simulink model "architecture"  (R2019a)
settings: Solver=VariableStepAuto  StartTime=0.0  StopTime=10.0  RelTol=1e-3
settings Model: Creator=gustavo.nunes  LastModifiedBy=gustavo.nunes

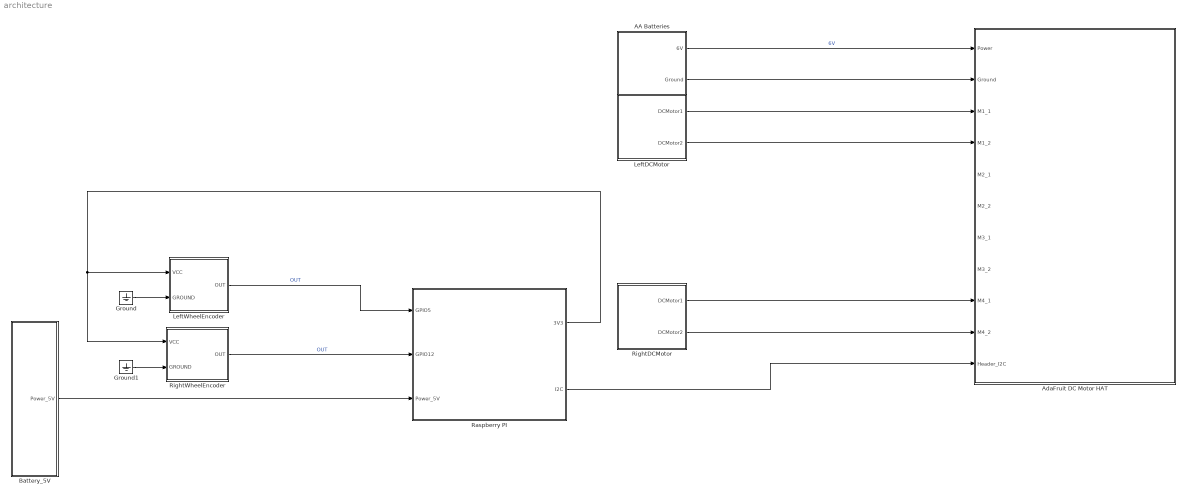
== system architecture ==
  AA Batteries : Subsystem
      mask Display: image('aa_battery.png');
  AdaFruit DC Motor HAT : Subsystem
  Battery_5V : Subsystem
      mask Display: image('battery.png');
  Ground : Ground
  Ground1 : Ground
  LeftDCMotor : Subsystem
      mask Display: image('tt_dc_motor.png');
  LeftWheelEncoder : Subsystem
      mask Display: image('wheel_encoder.png');
  Raspberry PI : Subsystem
  RightDCMotor : Subsystem
      mask Display: image('tt_dc_motor.png');
  RightWheelEncoder : Subsystem
      mask Display: image('wheel_encoder.png');
  wires:
  AA Batteries/1(6V) -> AdaFruit DC Motor HAT/1(Power)  "6V"
  AA Batteries/2(Ground) -> AdaFruit DC Motor HAT/2(Ground)
  Raspberry PI/2(I2C) -> AdaFruit DC Motor HAT/11(Header_I2C)
  LeftDCMotor/1(DCMotor1) -> AdaFruit DC Motor HAT/3(M1_1)
  LeftDCMotor/2(DCMotor2) -> AdaFruit DC Motor HAT/4(M1_2)
  RightDCMotor/1(DCMotor1) -> AdaFruit DC Motor HAT/9(M4_1)
  RightDCMotor/2(DCMotor2) -> AdaFruit DC Motor HAT/10(M4_2)
  Battery_5V/1(Power_5V) -> Raspberry PI/3(Power_5V)
  LeftWheelEncoder/1(OUT) -> Raspberry PI/1(GPIO5)  "OUT"
  RightWheelEncoder/1(OUT) -> Raspberry PI/2(GPIO12)  "OUT"
  Ground/1 -> LeftWheelEncoder/2(GROUND)
  Ground1/1 -> RightWheelEncoder/2(GROUND)
  Raspberry PI/1(3V3) -> RightWheelEncoder/1(VCC), LeftWheelEncoder/1(VCC)

== system architecture/AA Batteries ==
  6V : Outport
  Ground : Outport  Port=2

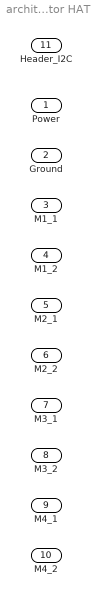
== system architecture/AdaFruit DC Motor HAT ==
  Power : Inport
  Ground : Inport  Port=2
  M1_1 : Inport  Port=3
  M1_2 : Inport  Port=4
  M2_1 : Inport  Port=5
  M2_2 : Inport  Port=6
  M3_1 : Inport  Port=7
  M3_2 : Inport  Port=8
  M4_1 : Inport  Port=9
  M4_2 : Inport  Port=10
  Header_I2C : Inport  Port=11

== system architecture/Battery_5V ==
  Power_5V : Outport

== system architecture/LeftDCMotor ==
  DCMotor1 : Outport
  DCMotor2 : Outport  Port=2

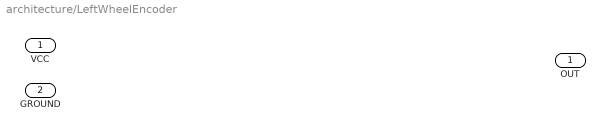
== system architecture/LeftWheelEncoder ==
  VCC : Inport
  GROUND : Inport  Port=2
  OUT : Outport

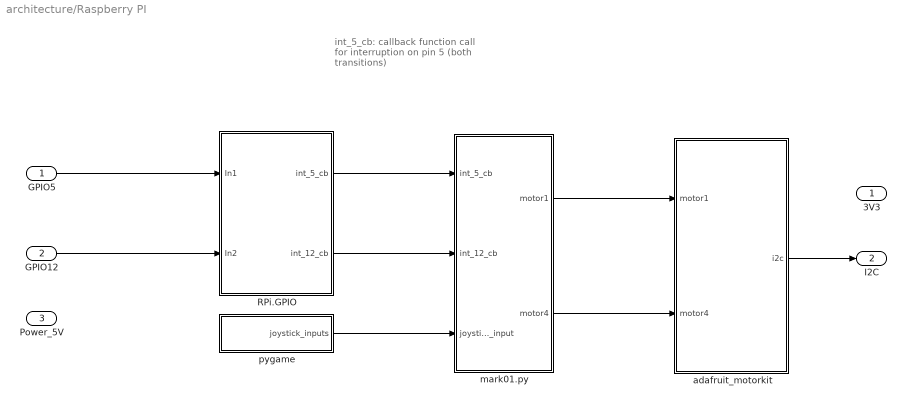
== system architecture/Raspberry PI ==
  note: int_5_cb: callback function call for interruption on pin 5 (both transitions)
  GPIO5 : Inport
  GPIO12 : Inport  Port=2
  Power_5V : Inport  Port=3
  RPi.GPIO : Subsystem
  adafruit_motorkit : Subsystem
  mark01.py : Subsystem
  pygame : Subsystem
  3V3 : Outport
  I2C : Outport  Port=2
  wires:
  adafruit_motorkit/1(i2c) -> I2C/1
  mark01.py/1(motor1) -> adafruit_motorkit/1(motor1)
  mark01.py/2(motor4) -> adafruit_motorkit/2(motor4)
  pygame/1(joystick_inputs) -> mark01.py/3(joystick_input)
  GPIO5/1 -> RPi.GPIO/1(In1)
  GPIO12/1 -> RPi.GPIO/2(In2)
  RPi.GPIO/1(int_5_cb) -> mark01.py/1(int_5_cb)
  RPi.GPIO/2(int_12_cb) -> mark01.py/2(int_12_cb)

== system architecture/RightDCMotor ==
  DCMotor1 : Outport
  DCMotor2 : Outport  Port=2

== system architecture/RightWheelEncoder ==
  VCC : Inport
  GROUND : Inport  Port=2
  OUT : Outport

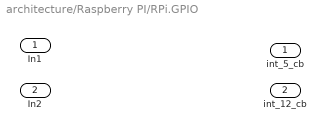
== system architecture/Raspberry PI/RPi.GPIO ==
  In1 : Inport
  In2 : Inport  Port=2
  int_5_cb : Outport
  int_12_cb : Outport  Port=2

== system architecture/Raspberry PI/adafruit_motorkit ==
  motor1 : Inport
  motor4 : Inport  Port=2
  i2c : Outport

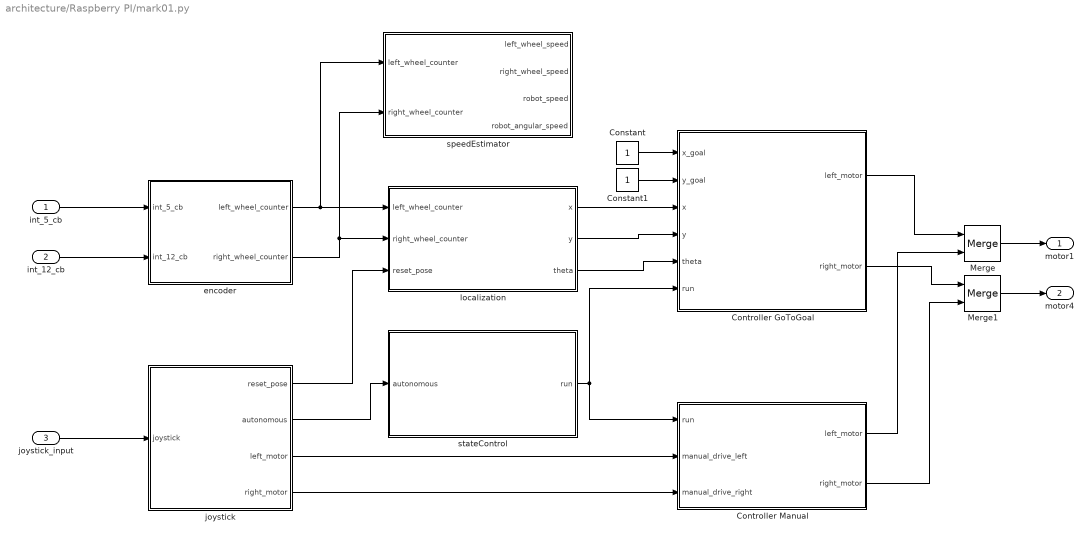
== system architecture/Raspberry PI/mark01.py ==
  int_5_cb : Inport
  int_12_cb : Inport  Port=2
  joystick_input : Inport  Port=3
  Constant : Constant
  Constant1 : Constant
  Controller GoToGoal : Subsystem
  Controller Manual : Subsystem
  Merge : Merge
  Merge1 : Merge
  encoder : Subsystem
  joystick : Subsystem
  localization : Subsystem
  speedEstimator : Subsystem
  stateControl : Subsystem
  motor1 : Outport
  motor4 : Outport  Port=2
  wires:
  int_5_cb/1 -> encoder/1(int_5_cb)
  int_12_cb/1 -> encoder/2(int_12_cb)
  joystick_input/1 -> joystick/1(joystick)
  encoder/1(left_wheel_counter) -> speedEstimator/1(left_wheel_counter), localization/1(left_wheel_counter)
  encoder/2(right_wheel_counter) -> speedEstimator/2(right_wheel_counter), localization/2(right_wheel_counter)
  joystick/1(reset_pose) -> localization/3(reset_pose)
  joystick/2(autonomous) -> stateControl/1(autonomous)
  Merge/1 -> motor1/1
  Merge1/1 -> motor4/1
  joystick/3(left_motor) -> Controller Manual/2(manual_drive_left)
  joystick/4(right_motor) -> Controller Manual/3(manual_drive_right)
  stateControl/1(run) -> Controller GoToGoal/6(run), Controller Manual/1(run)
  Controller GoToGoal/1(left_motor) -> Merge/1
  Controller GoToGoal/2(right_motor) -> Merge1/1
  Controller Manual/1(left_motor) -> Merge/2
  Controller Manual/2(right_motor) -> Merge1/2
  localization/1(x) -> Controller GoToGoal/3(x)
  localization/2(y) -> Controller GoToGoal/4(y)
  localization/3(theta) -> Controller GoToGoal/5(theta)
  Constant/1 -> Controller GoToGoal/1(x_goal)
  Constant1/1 -> Controller GoToGoal/2(y_goal)

== system architecture/Raspberry PI/pygame ==
  joystick_inputs : Outport

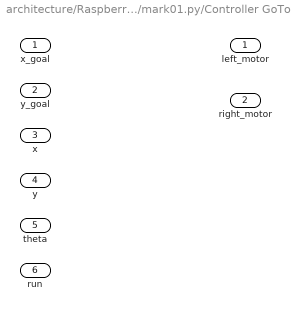
== system architecture/Raspberry PI/mark01.py/Controller GoToGoal ==
  x_goal : Inport
  y_goal : Inport  Port=2
  x : Inport  Port=3
  y : Inport  Port=4
  theta : Inport  Port=5
  run : Inport  Port=6
  left_motor : Outport
  right_motor : Outport  Port=2

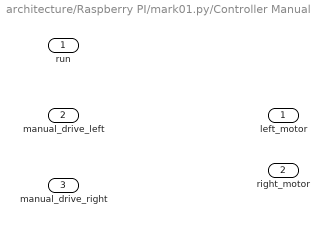
== system architecture/Raspberry PI/mark01.py/Controller Manual ==
  run : Inport
  manual_drive_left : Inport  Port=2
  manual_drive_right : Inport  Port=3
  left_motor : Outport
  right_motor : Outport  Port=2

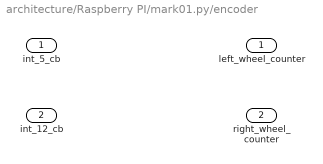
== system architecture/Raspberry PI/mark01.py/encoder ==
  int_5_cb : Inport
  int_12_cb : Inport  Port=2
  left_wheel_counter : Outport
  right_wheel_counter : Outport  Port=2

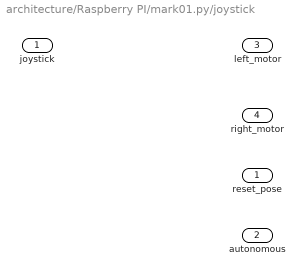
== system architecture/Raspberry PI/mark01.py/joystick ==
  joystick : Inport
  reset_pose : Outport
  autonomous : Outport  Port=2
  left_motor : Outport  Port=3
  right_motor : Outport  Port=4

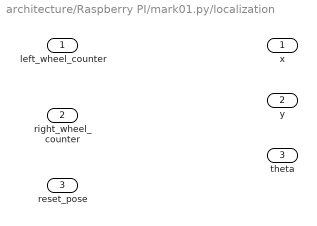
== system architecture/Raspberry PI/mark01.py/localization ==
  left_wheel_counter : Inport
  right_wheel_counter : Inport  Port=2
  reset_pose : Inport  Port=3
  x : Outport
  y : Outport  Port=2
  theta : Outport  Port=3

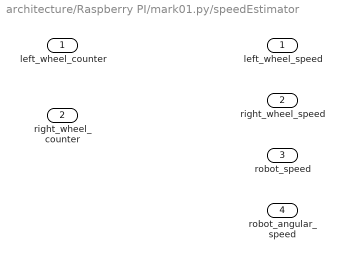
== system architecture/Raspberry PI/mark01.py/speedEstimator ==
  left_wheel_counter : Inport
  right_wheel_counter : Inport  Port=2
  left_wheel_speed : Outport
  right_wheel_speed : Outport  Port=2
  robot_speed : Outport  Port=3
  robot_angular_speed : Outport  Port=4

== system architecture/Raspberry PI/mark01.py/stateControl ==
  autonomous : Inport
  run : Outport
